simulink model "LKAS_AutoSave_20200908_1055"  (R2018b)
settings: Solver=FixedStepDiscrete  StartTime=0.0  StopTime=10.0  FixedStep=0.01  RelTol=1e-3
InitFcn:
  | tmpVer = ver('MATLAB');
  | tmpVer = str2num(tmpVer.Version);
  | % -------------------------------------------------------------------
  | %  MATLAB file generated by Simulink.saveVars on 21-Nov-2019 10:06:14
  | %  MATLAB version: 7.13.0.564 (R2011b)
  | % -------------------------------------------------------------------
  | 
  | 
  | SInt16 = Simulink.AliasType;
  | SInt16.Description = 'Num';
  | if (tmpVer > 7.11)
  | 	SInt16.DataScope = 'Auto';
  | end
  | SInt16.HeaderFile = 'Rte_Type.h';
  | SInt16.BaseType = 'int16';
  | 
  | SInt32 = Simulink.AliasType;
  | SInt32.Description = 'Num';
  | if (tmpVer > 7.11)
  | 	SInt32.DataScope = 'Auto';
  | end
  | SInt32.HeaderFile = 'Rte_Type.h';
  | SInt32.BaseType = 'int32';
  | 
  | SInt8 = Simulink.AliasType;
  | SInt8.Description = 'Num';
  | if (tmpVer > 7.11)
  | 	SInt8.DataScope = 'Auto';
  | end
  | SInt8.HeaderFile = 'Rte_Type.h';
  | SInt8.BaseType = 'int8';
  | 
  | T_A_m2_1024_1_u32 = Simulink.NumericType;
  | T_A_m2_1024_1_u32.Description = 'm2 (square meters  (m2))';
  | if (tmpVer > 7.11)
  | 	T_A_m2_1024_1_u32.DataScope = 'Auto';
  | end
  | T_A_m2_1024_1_u32.HeaderFile = 'Rte_Type.h';
  | T_A_m2_1024_1_u32.DataTypeMode = 'Fixed-point: slope and bias scaling';
  | T_A_m2_1024_1_u32.SignednessBool = false;
  | T_A_m2_1024_1_u32.WordLength = 32;
  | T_A_m2_1024_1_u32.FixedExponent = -10;
  | T_A_m2_1024_1_u32.SlopeAdjustmentFactor = 1;
  | T_A_m2_1024_1_u32.Bias = 0;
  | T_A_m2_1024_1_u32.DataTypeOverride = 'Inherit';
  | T_A_m2_1024_1_u32.IsAlias = true;
  | 
  | T_A_m2_65536_1_u16 = Simulink.NumericType;
  | T_A_m2_65536_1_u16.Description = 'm2 (square meters  (m2))';
  | if (tmpVer > 7.11)
  | 	T_A_m2_65536_1_u16.DataScope = 'Auto';
  | end
  | T_A_m2_65536_1_u16.HeaderFile = 'Rte_Type.h';
  | T_A_m2_65536_1_u16.DataTypeMode = 'Fixed-point: slope and bias scaling';
  | T_A_m2_65536_1_u16.SignednessBool = false;
  | T_A_m2_65536_1_u16.WordLength = 16;
  | T_A_m2_65536_1_u16.FixedExponent = -16;
  | T_A_m2_65536_1_u16.SlopeAdjustmentFactor = 1;
  | T_A_m2_65536_1_u16.Bias = 0;
  | T_A_m2_65536_1_u16.DataTypeOverride = 'Inherit';
  | ... (+4598 lines)
StopFcn:
  | clear  T_A_m2_1024_1_u32 T_A_m2_65536_1_u16 T_A_m2_Float32 T_A_mm2_10_1_u16 T_A_mm2_4_1_s16 T_A_mm2_Float32 T_Cnt_Num_10_1_u32 T_Cnt_Num_1_1_s16 T_Cnt_Num_1_1_s32 T_Cnt_Num_1_1_s8 T_Cnt_Num_1_1_u16 T_Cnt_Num_1_1_u32 T_Cnt_Num_1_1_u8 T_E_J_1_1_s32 T_E_J_Float32 T_E_kJ_128_1_s32 T_E_kJ_Float32 T_E_kwh_10_1_u16 T_E_kwh_Float32 T_Epl_kwhpkm_100_1_u16 T_Epl_kwhpkm_Float32 T_F_N_1_1_s16 T_F_N_Float32 T_I_A_1000_1_u16 T_I_A_1048576_1_s32 T_I_A_2048_1_s16 T_I_A_32_1_s16 T_I_A_Float32 T_I_mA_1_1_s16 T_I_mA_32768_128_s16 T_I_mA_Float32 T_J_kgpm2_128_1_u16 T_J_kgpm2_Float32 T_K_NA_1000_1_s16 T_K_NA_100_1_s16 T_K_NA_100_1_u16 T_K_NA_1024_1_s16 T_K_NA_1024_1_u16 T_K_NA_128_1_s16 T_K_NA_128_1_u16 T_K_NA_128_1_u8 T_K_NA_16777216_1_u32 T_K_NA_16_1_s16 T_K_NA_16_1_u16 T_K_NA_16_1_u8 T_K_NA_1_16_u16 T_K_NA_1_1_s16 T_K_NA_1_1_u16 T_K_NA_1_1_u8 T_K_NA_32768_1_s16 T_K_NA_32768_1_u16 T_K_NA_32_1_s8 T_K_NA_4096_1_u16 T_K_NA_4194304_1_s32 T_K_NA_4194304_1_u16 T_K_NA_65536_1_s32 T_K_NA_65536_1_u16 T_K_NA_8192_1_s16 T_K_NA_8_1_s16 T_K_NA_Float32 T_M_Nm_16_1_s16 T_M_Nm_1_1_s16 T_M_Nm_32768_1_s16 T_M_Nm_32_1_s16 T_M_Nm_4_1_s16 T_M_Nm_512_1_s16 T_M_Nm_Float32 T_P_W_1_4_s16 T_P_W_1_8_s16 T_P_W_Float32 T_P_kW_128_1_s16 T_P_kW_1_8_s16 T_P_kW_8_1_s32 T_P_kW_Float32 T_Pct_pct_1024_1_s32 T_Pct_pct_1024_1_u32 T_Pct_pct_10_1_s16 T_Pct_pct_10_1_u32 T_Pct_pct_128_100_s8 T_Pct_pct_1_1_s16 T_Pct_pct_1_4_u8 T_Pct_pct_255_100_u16 T_Pct_pct_255_100_u8 T_Pct_pct_256_1_s16 T_Pct_pct_256_1_u16 T_Pct_pct_65535_100_u16 T_Pct_pct_Float32 T_R_ohm_1024_1_s16 T_R_ohm_32_1_s16 T_R_ohm_Float32 T_TK_K_16_1_s16 T_TK_K_Float32 T_T_degC_10_400_1_u16 T_T_degC_16_1_s16 T_T_degC_1_40_1_u8 T_T_degC_2_80_1_u8 T_T_degC_Float32 T_U_V_1000_1_u16 T_U_V_10_1_u8 T_U_V_200_1_u8 T_U_V_32_1_s16 T_U_V_4096_1_s16 T_U_V_512_1_s16 T_U_V_65535_8_u16 T_U_V_8192_1_u16 T_U_V_Float32 T_U_mV_1_1_s16 T_U_mV_256_20_u16 T_U_mV_Float32 T_V_l_256_1_s16 T_V_l_4096_1_s16 T_V_l_64_1_s16 T_V_l_65535_100_u16 T_V_l_Float32 T_V_ml_128_1_s16 T_V_ml_1_1_s16 T_V_ml_32768_1_s16 T_V_ml_Float32 T_V_ul_32_1_u16 T_V_ul_Float32 T_Vpl_clpkm_512_1_u16 T_Vpl_clpkm_Float32 T_a_kphps_16_1_s16 T_a_kphps_Float32 T_a_mps2_128_1_s16 T_a_mps2_Float32 T_c_MJpkg_256_1_s16 T_c_MJpkg_Float32 T_c_kJpgpK_1024_1_s16 T_c_kJpgpK_Float32 T_c_kJpkgpK_128_1_u16 T_c_kJpkgpK_Float32 T_chrg_Ah_1_1_s16 T_chrg_Ah_1_1_u16 T_chrg_Ah_1_1_u8 T_chrg_Ah_256_1_u16 T_chrg_Ah_4194304_1_s32 T_chrg_Ah_512_1_u16 T_chrg_Ah_8_1_u16 T_chrg_Ah_Float32 T_cmp_NA_100_1_s16 T_cmp_NA_128_1_s16 T_cmp_NA_16_1_s16 T_cmp_NA_32768_1_u16 T_cmp_NA_Float32 T_d2n_rpmps2_4_1_s16 T_d2n_rpmps2_Float32 T_dPct_pctps_16_1_s16 T_dPct_pctps_256_1_s16 T_dPct_pctps_Float32 T_dT_degCps_128_1_s16 T_dT_degCps_Float32 T_dV_lph_1_1_s16 T_dV_lph_Float32 T_dV_lpm_128_1_s16 T_dV_lpm_32_1_s16 T_dV_lpm_Float32 T_dV_lps_1024_1_u16 T_dV_lps_4_1_u16 T_dV_lps_Float32 T_dV_mlps_1024_1_s16 T_dV_mlps_Float32 T_d_BitField16 T_dm_gps_128_1_s16 T_dm_gps_128_1_u16 T_dm_gps_256_1_u16 T_dm_gps_Float32 T_dm_mgps_1_1_s16 T_dm_mgps_Float32 T_dn_rpmps_1_1_s16 T_dn_rpmps_2_1_s16 T_dn_rpmps_Float32 T_dp_Paps_1_1_s16 T_dp_Paps_Float32 T_dp_kPaps_1_1_s16 T_dp_kPaps_8_1_s16 T_dp_kPaps_Float32 T_dphi_degps_128_1_s16 T_dphi_degps_8_1_s16 T_dphi_degps_Float32 T_dr_ps_256_1_s16 T_dr_ps_Float32 T_drho_mgplps_1_2_s16 T_drho_mgplps_Float32 T_e_NA_1_1_u8 T_f_Hz_1_1_u16 T_f_Hz_1_1_u32 T_f_Hz_64_1_u16 T_f_Hz_8_1_s16 T_f_Hz_Float32 T_g_BitField32 T_l_km_16_1_s16 T_l_km_1_1_u16 T_l_km_1_1_u32 T_l_km_Float32 T_l_m_1024_1_s16 T_l_m_16_1_s16 T_l_m_1_1_u32 T_l_m_Float32 T_l_mm_16_1_s16 T_l_mm_1_1_u16 T_l_mm_4096_1_s16 T_l_mm_4_1_u8 T_l_mm_64_1_s16 T_l_mm_Float32 T_m_g_1_1_s16 T_m_g_2048_1_s16 T_m_g_32_1_u16 T_m_g_Float32 T_m_kg_1024_1_s16 T_m_kg_1_1_s16 T_m_kg_1_1_u32 T_m_kg_Float32 T_m_mg_128_1_s16 T_m_mg_32_1_s16 T_m_mg_Float32 T_n_rpm_1_1_s16 T_n_rpm_1_25_u8 T_n_rpm_256_50_u16 T_n_rpm_2_25_u8 T_n_rpm_4_1_u16 T_n_rpm_Float32 T_p_MPa_64_1_s16 T_p_MPa_Float32 T_p_Pa_1_1_s16 T_p_Pa_Float32 T_p_kPa_1_10_u16 T_p_kPa_1_1_s16 T_p_kPa_1_1_u8 T_p_kPa_256_1_u16 T_p_kPa_32_1_u16 T_p_kPa_64_1_s16 T_p_kPa_Float32 T_phi_deg_100_1_s16 T_phi_deg_1024_1_s16 T_phi_deg_128_1_s16 T_phi_deg_1_1_u8 T_phi_deg_256_1_s16 T_phi_deg_2_1_s8 T_phi_deg_32_1_s16 T_phi_deg_512_6_s32 T_phi_deg_Float32 T_phi_rad_2048_1_s16 T_phi_rad_Float32 T_r_NA_1024_1_s16 T_r_NA_1024_1_u16 T_r_NA_16384_1_s16 T_r_NA_16_1_s16 T_r_NA_256_1_s8 T_r_NA_256_1_u16 T_r_NA_32768_1_u16 T_r_NA_32_1_u16 T_r_NA_4096_1_s16 T_r_NA_65535_2_u16 T_r_NA_8192_1_u16 T_r_NA_Float32 T_rho_gpl_8192_1_s16 T_rho_gpl_Float32 T_rho_kgpm3_16_1_s16 T_rho_kgpm3_Float32 T_rho_mgpl_1_1_s16 T_rho_mgpl_64_1_s16 T_rho_mgpl_Float32 T_t_hour_1_1_s16 T_t_hour_Float32 T_t_m_1_1_u16 T_t_m_Float32 T_t_ms_1_1_s16 T_t_ms_1_1_u16 T_t_ms_1_1_u32 T_t_ms_4096_1_s16 T_t_ms_64_1_s16 T_t_ms_Float32 T_t_s_1000_1_s16 T_t_s_100_1_s16 T_t_s_10_1_s16 T_t_s_10_1_u16 T_t_s_1_1_s16 T_t_s_1_1_u16 T_t_s_1_1_u32 T_t_s_Float32 T_t_us_10_1_u32 T_t_us_1_1_s16 T_t_us_1_1_u32 T_t_us_1_4_u16 T_t_us_Float32 T_v_kph_1_1_u8 T_v_kph_64_1_s16 T_v_kph_64_1_u16 T_v_kph_Float32 T_v_mps_256_1_s16 T_v_mps_Float32 T_w_radps_32_1_s16 T_w_radps_Float32 T_y_BitField8 T_y_BitFieldDiagProgress T_y_BitFieldDiagStatus T_y_NA_1_1_u8 SInt16 SInt32 SInt8 T_BOOLEAN UInt16 UInt32 UInt8 s16 s32 s8 u16 u32 u8
model workspace (MAT data in the model file):
  MCOS : class17 (value not decoded)
  MCOS : class17 (value not decoded)
  MCOS : class17 (value not decoded)
  MCOS : class17 (value not decoded)
  MCOS : class17 (value not decoded)
  MCOS : class17 (value not decoded)
  MCOS : class17 (value not decoded)
  MCOS : class17 (value not decoded)
  MCOS : class17 (value not decoded)
  MCOS : class17 (value not decoded)
  MCOS : class17 (value not decoded)
  MCOS : class17 (value not decoded)
  MCOS : class17 (value not decoded)
  MCOS : class17 (value not decoded)
  MCOS : class17 (value not decoded)
  MCOS : class17 (value not decoded)
  MCOS : class17 (value not decoded)
  MCOS : class17 (value not decoded)
  MCOS : class17 (value not decoded)
  MCOS : class17 (value not decoded)
  MCOS : class17 (value not decoded)
  MCOS : class17 (value not decoded)
  MCOS : class17 (value not decoded)
  MCOS : class17 (value not decoded)
  MCOS : class17 (value not decoded)
  MCOS : class17 (value not decoded)
  MCOS : class17 (value not decoded)
  MCOS : class17 (value not decoded)
  MCOS : class17 (value not decoded)
  MCOS : class17 (value not decoded)
  MCOS : class17 (value not decoded)
  MCOS : class17 (value not decoded)
  MCOS : class17 (value not decoded)
  MCOS : class17 (value not decoded)
  MCOS : class17 (value not decoded)
  MCOS : class17 (value not decoded)
  MCOS : class17 (value not decoded)
  MCOS : class17 (value not decoded)
  MCOS : class17 (value not decoded)
  MCOS : class17 (value not decoded)
  MCOS : class17 (value not decoded)
  MCOS : class17 (value not decoded)
  MCOS : class17 (value not decoded)
  MCOS : class17 (value not decoded)
  MCOS : class17 (value not decoded)
  MCOS : class17 (value not decoded)
  MCOS : class17 (value not decoded)
  MCOS : class17 (value not decoded)
  MCOS : class17 (value not decoded)
  MCOS : class17 (value not decoded)
  MCOS : class17 (value not decoded)
  MCOS : class17 (value not decoded)
  MCOS : class17 (value not decoded)
  MCOS : class17 (value not decoded)
  MCOS : class17 (value not decoded)
  MCOS : class17 (value not decoded)
  MCOS : class17 (value not decoded)
  MCOS : class17 (value not decoded)
  MCOS : class17 (value not decoded)
  MCOS : class17 (value not decoded)
  MCOS : class17 (value not decoded)
  MCOS : class17 (value not decoded)
  MCOS : class17 (value not decoded)
  MCOS : class17 (value not decoded)
  MCOS : class17 (value not decoded)
  MCOS : class17 (value not decoded)
  MCOS : class17 (value not decoded)
  MCOS : class17 (value not decoded)
  MCOS : class17 (value not decoded)
  MCOS : class17 (value not decoded)
  MCOS : class17 (value not decoded)
  MCOS : class17 (value not decoded)
  MCOS : class17 (value not decoded)
  MCOS : class17 (value not decoded)
  MCOS : class17 (value not decoded)
  MCOS : class17 (value not decoded)
  MCOS : class17 (value not decoded)
  MCOS : class17 (value not decoded)
  MCOS : class17 (value not decoded)
  MCOS : class17 (value not decoded)
  MCOS : class17 (value not decoded)
  MCOS : class17 (value not decoded)
  MCOS : class17 (value not decoded)
  MCOS : class17 (value not decoded)
  MCOS : class17 (value not decoded)
  MCOS : class17 (value not decoded)
  MCOS : class17 (value not decoded)
  MCOS : class17 (value not decoded)
  MCOS : class17 (value not decoded)
undefined symbols (not defined in the file): LKA_CarWidth, LKA_SampleTime, LKA_StrRatio_C, LKA_Veh2CamL_C, LKA_Veh2CamW_C, LKA_WhlBaseL_C, LL_CompSWA_C, LL_CrvtPrvwT_C, LL_DesDvt_C, LL_DvtComp_C, LL_DvtPrvwT_C, LL_DvtSpdDet_vDvtSpdMin_C, LL_HdAgExT_C, LL_HdAgPrvwT_C, LL_LAccMax_C, LL_LAccRMax_C, LL_LDW_EarliestWarnLine_C, LL_LDW_LatestWarnLine_C, LL_LDWS_SUPPRESS_HEADING, LL_LFClb_TFC_DiffCtlBalance, LL_LFClb_TFC_DiffCtrlMaxSWA, LL_LFClb_TFC_DiffCtrlRatio, LL_LFClb_TFC_facmGainLutGain1_C, LL_LFClb_TFC_facmGainLutGain2_C, LL_LFClb_TFC_facmIntegRatio, LL_LFClb_TFC_facmKlat_C, LL_LFClb_TFC_FfCtlRatio_C, LL_LFClb_TFC_phiIntegCtlMaxSWA_C, LL_LFClb_TFC_tiKlatPrvwT_C, LL_LFClb_TFC_vGainLutVehSpdLwr_C, LL_LFClb_TFC_vGainLutVehSpdUpr_C, LL_LKA_EarliestWarnLine_C, LL_LKA_LatestWarnLine_C, LL_LKAExPrcs_ExitC0Dvt, LL_LKAExPrcs_ExitC0Swt, LL_LKAExPrcs_tiExitTime1, LL_LKAExPrcs_tiExitTime2, LL_LKAExPrcs_tiExitTime3, LL_LKAS_OUT_OF_CONTROL_LAT_VEL, LL_LKAS_OUT_OF_CONTROL_TTLC, LL_LKASWASyn_M0, LL_LKASWASyn_M1, LL_LKASWASyn_M2, LL_LKASWASyn_M3K, LL_LKASWASyn_SWAaddMax, LL_LKASWASyn_T2, LL_LKASWASyn_tiTrqSwaRtTime, LL_LKASWASyn_tiTrqSwaTime, LL_LKASWASyn_TrqMax, LL_LKASWASyn_TrqSwaAddSwt, LL_LKASWASyn_TrqSwaRateDiff, LL_LSpdCompT_C, LL_lStpLngth_C, LL_MAX_DELAY_EPSSTAR_TIME, LL_MAX_DRIVER_TORQUE_DISABLE, LL_MAX_DRIVER_TORQUE_ENABLE, LL_MAX_LANE_WIDTH_DISABLE, LL_MAX_LANE_WIDTH_ENABLE, LL_MAX_LAT_ACC_DISABLE, LL_MAX_LAT_ACC_ENABLE ... (+29)
libraries: simulink x134, dspstat3 x3, simulink_extras x1
(part 6 of 19)

== system LKAS_AutoSave_20200908_1055/LKAS/LL/LL Inputs Mapping/bsVehMovInfo ==
  bsVehMovInfoIn : Inport
  Bus Creator : BusCreator  Inputs=10
  Bus Selector2 : BusSelector  OutputSignals=ESC_LatAcc,ESC_LatAcc_Valid,ESC_YawRate,ESC_YawRate_Valid,ESC_UnYawRate,ESC_VehSpd,ESC_LonAcc,ESC_LonAcc_Valid,ESC_Brake_Press,ESC_VehSpd_Valid
  bsVehMovInfoOut : Outport
  wires:
  Bus Creator/1 -> bsVehMovInfoOut/1
  Bus Selector2/10 -> Bus Creator/10  "<ESC_VehSpd_Valid>"
  Bus Selector2/9 -> Bus Creator/9  "<ESC_Brake_Press>"
  Bus Selector2/8 -> Bus Creator/8  "<ESC_LonAcc_Valid>"
  Bus Selector2/7 -> Bus Creator/7  "<ESC_LonAcc>"
  Bus Selector2/6 -> Bus Creator/6  "<ESC_VehSpd>"
  Bus Selector2/5 -> Bus Creator/5  "<ESC_UnYawRate>"
  Bus Selector2/4 -> Bus Creator/4  "<ESC_YawRate_Valid>"
  Bus Selector2/3 -> Bus Creator/3  "<ESC_YawRate>"
  Bus Selector2/2 -> Bus Creator/2  "<ESC_LatAcc_Valid>"
  Bus Selector2/1 -> Bus Creator/1  "<ESC_LatAcc>"
  bsVehMovInfoIn/1 -> Bus Selector2/1

== system LKAS_AutoSave_20200908_1055/LKAS/LL/LLOn/LDW ==
  LDW_stLDWActvFlg : Inport
  LDW_bsInInfoSyn : Inport  Port=2
  LDW_bsLDWClb : Inport  Port=3
  states : EnablePort  StatesWhenEnabling=reset
      settings: AttributesFormatString=states = %<StatesWhenEnabling>
  Bus Selector : BusSelector  OutputSignals=bsLaneInfo.bsL0Info.L0_C1,bsLaneInfo.bsR0Info.R0_C1
  Bus Selector1 : BusSelector  OutputSignals=LL_LDWS_SUPPRESS_HEADING
  Heading Angle Detection (HdAgDet) : Subsystem  Description=|
      | Block Name: Heading Angle Detection
      | Ab.: HdAgDet
      | No.: 1.3.1.0
      | Rev: 0.0.1
      | Update Date: 19-3-26
  LDWWarnInfo : MATLAB Function  TreatAsAtomicUnit=on
  LDW_Flag : Outport  OutputWhenDisabled=reset  InitialOutput=0
  wires:
  LDW_bsInInfoSyn/1 -> Bus Selector/1
  LDW_stLDWActvFlg/1 -> Heading Angle Detection (HdAgDet)/1(HdAgDet_stLDWActvFlg), LDWWarnInfo/1(LDW_stLDWActvFlg)
  Bus Selector/1 -> Heading Angle Detection (HdAgDet)/2(HdAgDet_phiHdAgLft)  "<L0_C1>"
  Bus Selector/2 -> Heading Angle Detection (HdAgDet)/3(HdAgDet_phiHdAgRgt)  "<R0_C1>"
  LDW_bsLDWClb/1 -> Bus Selector1/1
  Bus Selector1/1 -> Heading Angle Detection (HdAgDet)/4(HdAgDet_phiHdAgThres_C)  "<LL_LDWS_SUPPRESS_HEADING>"
  Heading Angle Detection (HdAgDet)/1(HdAgDet_stHdAgDetFlg) -> LDWWarnInfo/2(LDW_stHdAgDetFlg)
  LDWWarnInfo/1(LDWWarnInfo) -> LDW_Flag/1

== system LKAS_AutoSave_20200908_1055/LKAS/LL/LLOn/LKA ==
  LKA_bsInInfoSyn : Inport
  LKA_bsLKAInPInfo : Inport  Port=2
  LKA_bsLKAClb : Inport  Port=3
  LKA_bsConstantClb : Inport  Port=4
  states = reset : EnablePort  StatesWhenEnabling=reset  ShowOutputPort=on
  Bus Selector : BusSelector  OutputSignals=LKA_SampleTime
  Cast To Single : DataTypeConversion  OutDataTypeStr=uint8
  Driver Torque Addition (DTA) : Subsystem
  LKA Exit Processing (LKAExPrcs) : Subsystem  Description=|
      | Block Name: LKA Exit Processing 
      | Ab.: LKAExPrcs
      | No.: 1.2.2.0
      | Rev: 0.0.1
      | Update Date: 19-5-13
  "LKA Motion Planning (LKAMP) " : Subsystem  Description=|
      | Block Name: LKA Motion Planning
      | Ab.: LKAMP
      | No.: 1.2.3.0
      | Rev: 0.0.1
      | Update Date: 19-5-13
  LKA SWA Limit (LKASWALim) : Subsystem  Description=|
      | Block Name: LKA SWA Synthesis
      | Ab.: LKASWASyn
      | No.: 1.2.6.0
      | Rev: 0.0.1
      | Update Date: 19-5-13
  LKA_Mon : Subsystem
  Lane Following (LF) : Subsystem  Description=|
      | Block Name: Lane Following
      | Ab.: LF
      | No.: 02
      | Rev: 00.00.01
      | Update Date: 19-3-28
  Plan To LaneFollowing (PTLF) : Subsystem
  LKA_ExitFlg : Outport  OutputWhenDisabled=reset  InitialOutput=0
  LKA_phiSWACmd : Outport  Port=2  OutputWhenDisabled=reset  InitialOutput=0
  LKA_M : Outport  Port=3  OutputWhenDisabled=reset  InitialOutput=0
  LKAMon : Outport  Port=4  OutputWhenDisabled=reset  InitialOutput=0
  tag scope: ActFlg=global, Ff=global, LKA_ConstantClb=global, LKA_ExitFlg_Mon=global, LKA_SampleTime=global, PT1=global
  wires:
  Bus Selector/1 -> [LKA_SampleTime]  "<LKA_SampleTime>"
  LKA_bsConstantClb/1 -> Bus Selector/1, [LKA_ConstantClb]
  Cast To Single/1 -> [ActFlg]  "ActFlg"
  Plan To LaneFollowing (PTLF)/1(SWACmd) -> LKA SWA Limit (LKASWALim)/1(LKASWALim_phiTFCSWACmd)  "PTLFSWACmd"
  states = reset/1 -> Cast To Single/1
  LKA SWA Limit (LKASWALim)/1(LKASWALim_phiSWACmd) -> LKA_phiSWACmd/1  "phiSWACmd"
  LKA Exit Processing (LKAExPrcs)/1(LKAExPrcs_stExFlg) -> [LKA_ExitFlg_Mon], LKA_ExitFlg/1
  [Ff] -> Plan To LaneFollowing (PTLF)/5(Ff)
  [P] -> Plan To LaneFollowing (PTLF)/6(P)
  [I] -> Plan To LaneFollowing (PTLF)/7(I)
  [D] -> Plan To LaneFollowing (PTLF)/8(D)
  Driver Torque Addition (DTA)/1(DTA_phiDTASWACmd) -> [DT]  "DT"
  [DT] -> Plan To LaneFollowing (PTLF)/4(DrvTrq)
  [Plan] -> Plan To LaneFollowing (PTLF)/2(Plan)
  [PT1] -> Plan To LaneFollowing (PTLF)/3(T1)
  [PT1] -> LKA Exit Processing (LKAExPrcs)/4(LKAExPrcs_PlanT1)
  [ActFlg] -> "LKA Motion Planning (LKAMP) "/2(LKAMP_stLKAActvFlg)
  [LKA_ConstantClb] -> "LKA Motion Planning (LKAMP) "/5(LLClb_bsConstantClb)
  [LKA_ConstantClb] -> Lane Following (LF)/4(LF_bsConstantClb)
  LKA_bsLKAInPInfo/1 -> [LKAInPInfo]
  [LKAInPInfo] -> "LKA Motion Planning (LKAMP) "/3(LKAMP_bsLKAInPInfo)
  [LKAInPInfo] -> LKA Exit Processing (LKAExPrcs)/2(LKAExPrcs_bsLKAInPInfo)
  [LKAInPInfo] -> Plan To LaneFollowing (PTLF)/1(InP)
  LKA_bsLKAClb/1 -> [LKA_bsLKAClb]
  [LKAInPInfo] -> LKA SWA Limit (LKASWALim)/3(LKASWALim_bsLKAInPInfo)
  [LKA_bsLKAClb] -> LKA Exit Processing (LKAExPrcs)/3(LKAExPrcs_bsLKAClb)
  [LKA_bsLKAClb] -> "LKA Motion Planning (LKAMP) "/4(LKAMP_bsLKAClb)
  [LKA_bsLKAClb] -> Driver Torque Addition (DTA)/2(DTA_bsLFClb)
  [LKA_bsLKAClb] -> Lane Following (LF)/3(LF_bsLFClb)
  [LKA_bsLKAClb] -> LKA SWA Limit (LKASWALim)/4(LKASWALim_bsLKAClb)
  LKA_bsInInfoSyn/1 -> [LKA_bsInInfoSyn]
  [LKA_bsInInfoSyn] -> LKA Exit Processing (LKAExPrcs)/1(LKAExPrcs_bsInInfoSyn)
  [LKA_bsInInfoSyn] -> "LKA Motion Planning (LKAMP) "/1(LKAMP_bsInInfoSyn)
  [LKA_bsInInfoSyn] -> Driver Torque Addition (DTA)/1(DTA_bsInInfoSyn)
  [LKA_bsInInfoSyn] -> Lane Following (LF)/1(LF_bsInInfoSyn)
  [Ff] -> LKA SWA Limit (LKASWALim)/2(LKASWALim_Ff)
  [LKAInPInfo] -> Lane Following (LF)/2(LF_bsLKAInPInfo)
  Driver Torque Addition (DTA)/2(DTA_M) -> LKA_M/1
  Lane Following (LF)/3(LF_phiIntegSWACmd) -> [I]
  Lane Following (LF)/1(LF_phiFfLFSWACmd) -> [Ff]
  Lane Following (LF)/2(LF_phiPropSWACmd) -> [P]
  Lane Following (LF)/4(LF_phiDiffSWACmd) -> [D]
  "LKA Motion Planning (LKAMP) "/1(LKAMP_phiSWACmd) -> [Plan]  "PlanSWACmd"
  "LKA Motion Planning (LKAMP) "/3(LKAMP_tiT2) -> ?  "PlanT2"
  "LKA Motion Planning (LKAMP) "/2(LKAMP_tiT1) -> [PT1]  "PlanT1"
  LKA_Mon/1(LKAMon) -> LKAMon/1

== system LKAS_AutoSave_20200908_1055/LKAS/LL/LLOn/LKA Input Processing (LKAInP) ==
  LKAInP_stLKAActvFlg : Inport
  LKAInP_bsInInfoSyn : Inport  Port=2
  LKAInP_bsLKAClb : Inport  Port=3
  Bus Creator : BusCreator  Inputs=6
  Bus Creator1 : BusCreator  Inputs=3
  Delay : Delay  DelayLength=1
  Lane Width Calculation (LW) : Subsystem
  Predicted Deviation Calculation (PrDvt) : Subsystem
  Predicted Heading Angle Calculation (PrHdAg) : Subsystem
  Previewed Curvature (PrCrvt) : Subsystem
  Steering Wheel Position Calculation (SWAPosCal) : Subsystem
  TTLC Calculation (TTLCCalc) : Subsystem  Description=|
      | Block Name: TTLC Calculation
      | Ab.: TTLCCalc
      | No.: 1.1.1.1
      | Rev: 0.0.1
      | Update Date: 19-3-26
  Under The Limit (UndrLim) : Subsystem
  LKAInP_bsLKAInPInfo : Outport
  wires:
  Delay/1 -> Previewed Curvature (PrCrvt)/1(PrvwCrvt_stLKAActvFlg), Predicted Heading Angle Calculation (PrHdAg)/2(PrdcHdAg_stLKAActvFlg), Predicted Deviation Calculation (PrDvt)/1(PrdcDvt_stLKAActvFlg)
  LKAInP_bsInInfoSyn/1 -> Steering Wheel Position Calculation (SWAPosCal)/1(SWAPosCal_bsInInfoSyn), Under The Limit (UndrLim)/1(UndrLim_bsInInfoSyn), Previewed Curvature (PrCrvt)/2(PrvwCrvt_bsInInfoSyn), Predicted Heading Angle Calculation (PrHdAg)/3(PrHdAg_bsInInfoSyn), Predicted Deviation Calculation (PrDvt)/2(PrdcDvt_bsInInfoSyn), TTLC Calculation (TTLCCalc)/1(bsInfo), Lane Width Calculation (LW)/1(LW_bsInInfoSyn)
  Bus Creator/1 -> LKAInP_bsLKAInPInfo/1
  LKAInP_bsLKAClb/1 -> Under The Limit (UndrLim)/2(UndrLim_bsUndrLimClb), Previewed Curvature (PrCrvt)/3(PrvwCrvt_tiCrvtPrvwT_C), Predicted Heading Angle Calculation (PrHdAg)/4(PrHdAg_bsLKAClb), Predicted Deviation Calculation (PrDvt)/4(PrdcDvt_bsLKAClb)
  Predicted Heading Angle Calculation (PrHdAg)/1(PrHdAg_bsPrHdAgInfo) -> Predicted Deviation Calculation (PrDvt)/3(PrdcDvt_bsPrdcHdAgInfo), Bus Creator1/2  "bsPrHdAgInfo"
  Predicted Deviation Calculation (PrDvt)/1(PrdcDvt_bsPrdcDvtInfo) -> TTLC Calculation (TTLCCalc)/2(bsPrDvtInfo), Bus Creator1/1  "bsPrDvtInfo"
  Previewed Curvature (PrCrvt)/1(PrvwCrvt_bsPrvwCrvtInfo) -> TTLC Calculation (TTLCCalc)/3(bsPrvwCrvtInfo), Bus Creator1/3  "bsPrCrvtInfo"
  Bus Creator1/1 -> Bus Creator/3  "Pr_bsPrInfo"
  Under The Limit (UndrLim)/1(UndrLim_phiSWAMax) -> Bus Creator/4  "UndrLim_phiSWAMax"
  Under The Limit (UndrLim)/2(UndrLim_dphiSWARMax) -> Bus Creator/5  "UndrLim_dphiSWARMax"
  LKAInP_stLKAActvFlg/1 -> Delay/1
  Steering Wheel Position Calculation (SWAPosCal)/1(SWAPosCal) -> Bus Creator/6  "LKAInP_phiSWAPos"
  Lane Width Calculation (LW)/1(LW_LaneWidth) -> Bus Creator/1  "LW_LaneWidth"
  TTLC Calculation (TTLCCalc)/1(TTLCCalc_bsTTLCInfo) -> Bus Creator/2, Predicted Heading Angle Calculation (PrHdAg)/1(PrHdAg_bsTTLCInfo)  "TTLC_bsTTLCInfo"

== system LKAS_AutoSave_20200908_1055/LKAS/LL/LLOn/LL State Determination (LLStateDet) ==
  LLStateDet_stDACMode : Inport
  LLStateDet_bsInInfoSyn : Inport  Port=2
  LLStateDet_bsLKAInPInfo : Inport  Port=3
  LLStateDet_bsLLSMConClb : Inport  Port=4
  LLStateDet_stExitFlg : Inport  Port=5
  LLStateDet_SignalFault : Inport  Port=6
  Bus Creator : BusCreator  Inputs=3
  Delay : Delay  DelayLength=1
  Delay1 : Delay  DelayLength=1
  LDW_State_Machine : Stateflow chart  Description=|  TreatAsAtomicUnit=on
      | Block Name: LDW State Machine
      | Ab.: LDWSM
      | No.: 1.1.2.0
      | Rev: 0.0.1
      | Update Date: 19-3-26
      settings: RTWSystemCode=Nonreusable function
  LKA_State_Machine : Stateflow chart  Description=|  TreatAsAtomicUnit=on
      | Block Name: LKA State Machine
      | Ab.: LKASM
      | No.: 1.1.3.0
      | Rev: 0.0.1
      | Update Date: 19-3-26
      settings: RTWSystemCode=Nonreusable function
  LL State Machine Conditions (LLSMCon) : Subsystem
  LLStateDet_bsLLState : Outport
  LLStateDet_stLDWActvFlg : Outport  Port=2
  LLStateDet_stLKAActvFlg : Outport  Port=3
  tag scope: LDW_State_Mon=global, LKA_State_Mon=global
  wires:
  LL State Machine Conditions (LLSMCon)/2(LLSMCon_stLDWEnaCSyn) -> LDW_State_Machine/2(LDWSM_stEnaCSyn)
  LL State Machine Conditions (LLSMCon)/3(LLSMCon_stLDWDisblCSyn) -> LDW_State_Machine/3(LDWSM_stDisblCSyn)
  LL State Machine Conditions (LLSMCon)/4(LLSMCon_stLDWActvCSyn) -> LDW_State_Machine/4(LDWSM_stActvCSyn)
  LL State Machine Conditions (LLSMCon)/5(LLSMCon_stLDWDeactvCSyn) -> LDW_State_Machine/5(LDWSM_stDeactvCSyn)
  LL State Machine Conditions (LLSMCon)/1(LLSMCon_stDACMode) -> LKA_State_Machine/1(LKASM_stLMCMode), Bus Creator/2, LDW_State_Machine/1(LDWSM_stLMCMode)  "DACMode"
  LDW_State_Machine/1(LDWSM_stLDWActvFlg) -> LLStateDet_stLDWActvFlg/1
  LKA_State_Machine/1(LKASM_stLKAActvFlg) -> LLStateDet_stLKAActvFlg/1
  Delay1/1 -> LL State Machine Conditions (LLSMCon)/5(LLSMCon_bsLLState)
  Bus Creator/1 -> Delay1/1, LLStateDet_bsLLState/1  "LLState"
  LKA_State_Machine/2(LKASM_stLKAState) -> [LKA_State_Mon], Bus Creator/3  "LKA_State"
  LDW_State_Machine/2(LDWSM_stLDWState) -> [LDW_State_Mon], Bus Creator/1  "LDW_State"
  LL State Machine Conditions (LLSMCon)/6(LLSMCon_stLDWFaultCSyn) -> LDW_State_Machine/6(LDWSM_stFaultCSyn)
  LL State Machine Conditions (LLSMCon)/7(LLSMCon_stLKAEnaCSyn) -> LKA_State_Machine/2(LKASM_stEnaCSyn)
  LL State Machine Conditions (LLSMCon)/8(LLSMCon_stLKADisblCSyn) -> LKA_State_Machine/3(LKASM_stDisblCSyn)
  LL State Machine Conditions (LLSMCon)/9(LLSMCon_stLKAActvCSyn) -> LKA_State_Machine/4(LKASM_stActvCSyn)
  LL State Machine Conditions (LLSMCon)/10(LLSMCon_stLKADeactvCSyn) -> LKA_State_Machine/5(LKASM_stDeactvCSyn)
  LL State Machine Conditions (LLSMCon)/11(LLSMCon_stLKAFaultCSyn) -> LKA_State_Machine/6(LKASM_stFaultCSyn)
  LLStateDet_bsInInfoSyn/1 -> LL State Machine Conditions (LLSMCon)/2(LLSMCon_bsInInfoSyn)
  LLStateDet_bsLKAInPInfo/1 -> LL State Machine Conditions (LLSMCon)/3(LLSMCon_bsLKAInPInfo)
  LLStateDet_stDACMode/1 -> LL State Machine Conditions (LLSMCon)/1(LLSMCon_stDACModeIn)
  LLStateDet_stExitFlg/1 -> Delay/1
  LLStateDet_bsLLSMConClb/1 -> LL State Machine Conditions (LLSMCon)/4(LLSMCon_bsLLSMConClb)
  Delay/1 -> LL State Machine Conditions (LLSMCon)/6(LLSMCon_stExitFlg)
  LLStateDet_SignalFault/1 -> LL State Machine Conditions (LLSMCon)/7(LLSMCon_bsSignalFault)

== system LKAS_AutoSave_20200908_1055/LKAS/LL/LLOn/LL_Mon ==
  LKAMon : Inport
  Bus : BusCreator  Inputs=3
  BusInP : BusCreator  Inputs=2
  BusState : BusCreator  Inputs=2
  LLMon : Outport
  wires:
  [InPMon] -> Bus/1
  [StateMon] -> Bus/2
  LKAMon/1 -> Bus/3
  Bus/1 -> LLMon/1  "LLMon"
  [LFTTTLC_Mon] -> BusInP/1  "LFTTTLC_Mon"
  [RGTTTLC_Mon] -> BusInP/2  "RGTTTLC_Mon"
  [LDW_State_Mon] -> BusState/1  "LDW_State_Mon"
  [LKA_State_Mon] -> BusState/2  "LKA_State_Mon"
  BusInP/1 -> [InPMon]  "InPMon"
  BusState/1 -> [StateMon]  "StateMon"

== system LKAS_AutoSave_20200908_1055/LKAS/LLClb/LLSMConClb/ICv to v ==
  In1 : Inport
  Add : Sum  Inputs=+-
  Constant : Constant  Value=2.5  OutDataTypeStr=single
  Gain : Gain  Gain=1/1.02
  Out1 : Outport
  wires:
  In1/1 -> Add/1
  Add/1 -> Gain/1
  Constant/1 -> Add/2
  Gain/1 -> Out1/1

== system LKAS_AutoSave_20200908_1055/LKAS/LLClb/LLSMConClb/ICv to v1 ==
  In1 : Inport
  Add : Sum  Inputs=+-
  Constant : Constant  Value=2.5  OutDataTypeStr=single
  Gain : Gain  Gain=1/1.02
  Out1 : Outport
  wires:
  Gain/1 -> Out1/1
  Constant/1 -> Add/2
  Add/1 -> Gain/1
  In1/1 -> Add/1

== system LKAS_AutoSave_20200908_1055/LKAS/LLClb/LLSMConClb/ICv to v2 ==
  In1 : Inport
  Add : Sum  Inputs=+-
  Constant : Constant  Value=2.5  OutDataTypeStr=single
  Gain : Gain  Gain=1/1.02
  Out1 : Outport
  wires:
  In1/1 -> Add/1
  Add/1 -> Gain/1
  Constant/1 -> Add/2
  Gain/1 -> Out1/1

== system LKAS_AutoSave_20200908_1055/LKAS/LLClb/LLSMConClb/ICv to v3 ==
  In1 : Inport
  Add : Sum  Inputs=+-
  Constant : Constant  Value=2.5  OutDataTypeStr=single
  Gain : Gain  Gain=1/1.02
  Out1 : Outport
  wires:
  Gain/1 -> Out1/1
  Constant/1 -> Add/2
  Add/1 -> Gain/1
  In1/1 -> Add/1

== system LKAS_AutoSave_20200908_1055/LKAS/LLClb/LLSMConClb/ICv to v4 ==
  In1 : Inport
  Add : Sum  Inputs=+-
  Constant : Constant  Value=2.5  OutDataTypeStr=single
  Gain : Gain  Gain=1/1.02
  Out1 : Outport
  wires:
  In1/1 -> Add/1
  Add/1 -> Gain/1
  Constant/1 -> Add/2
  Gain/1 -> Out1/1

== system LKAS_AutoSave_20200908_1055/LKAS/LLClb/LLSMConClb/ICv to v5 ==
  In1 : Inport
  Add : Sum  Inputs=+-
  Constant : Constant  Value=2.5  OutDataTypeStr=single
  Gain : Gain  Gain=1/1.02
  Out1 : Outport
  wires:
  Gain/1 -> Out1/1
  Constant/1 -> Add/2
  Add/1 -> Gain/1
  In1/1 -> Add/1

== system LKAS_AutoSave_20200908_1055/LKAS/LL/Human Machine Interface (HMI)/Subsystem/Count 10s ==
  Enable : EnablePort  StatesWhenEnabling=reset
  Add : Sum
  Compare To Constant27 : simulink/Logic and Bit Operations/Compare To Constant  relop=>=  const=1000  OutDataTypeStr=boolean
  Constant : Constant  OutDataTypeStr=uint16
  Memory : Memory  InheritSampleTime=on
  Saturation : Saturate  UpperLimit=2100  LowerLimit=0
  Out : Outport  OutputWhenDisabled=reset  InitialOutput=0
  wires:
  Memory/1 -> Add/2
  Saturation/1 -> Memory/1, Compare To Constant27/1
  Add/1 -> Saturation/1
  Constant/1 -> Add/1
  Compare To Constant27/1 -> Out/1

== system LKAS_AutoSave_20200908_1055/LKAS/LL/Human Machine Interface (HMI)/Subsystem/Count 15s ==
  Enable : EnablePort  StatesWhenEnabling=reset
  Add : Sum
  Compare To Constant27 : simulink/Logic and Bit Operations/Compare To Constant  relop=>=  const=1500  OutDataTypeStr=boolean
  Constant : Constant  OutDataTypeStr=uint16
  Memory : Memory  InheritSampleTime=on
  Saturation : Saturate  UpperLimit=2100  LowerLimit=0
  Out : Outport  OutputWhenDisabled=reset  InitialOutput=0
  wires:
  Compare To Constant27/1 -> Out/1
  Constant/1 -> Add/1
  Add/1 -> Saturation/1
  Saturation/1 -> Compare To Constant27/1, Memory/1
  Memory/1 -> Add/2

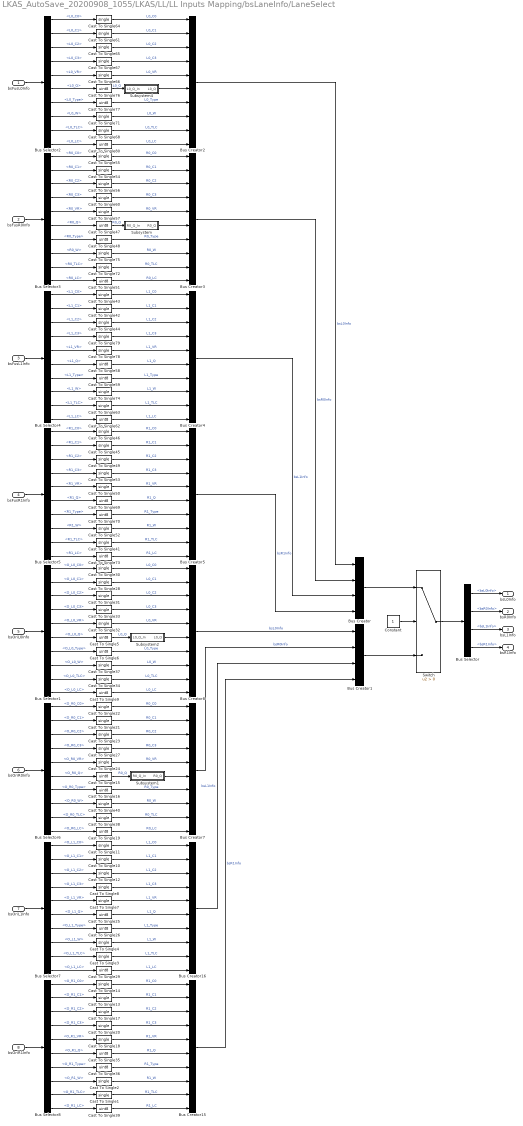
== system LKAS_AutoSave_20200908_1055/LKAS/LL/LL Inputs Mapping/bsLaneInfo/LaneSelect ==
  bsFusL0Info : Inport
  bsFusR0Info : Inport  Port=2
  bsFusL1Info : Inport  Port=3
  bsFusR1Info : Inport  Port=4
  bsOriL0Info : Inport  Port=5
  bsOriR0Info : Inport  Port=6
  bsOriL1Info : Inport  Port=7
  bsOriR1Info : Inport  Port=8
  Bus Creator : BusCreator  Inputs=4
  Bus Creator1 : BusCreator  Inputs=4
  Bus Creator{2..5,7..8,15..16} (8 alike) : BusCreator  Inputs=10
  Bus Selector : BusSelector  OutputSignals=bsL0Info,bsR0Info,bsL1Info,bsR1Info
  Bus Selector1 : BusSelector  OutputSignals=O_L0_C0,O_L0_C1,O_L0_C2,O_L0_C3,O_L0_VR,O_L0_Q,O_L0_Type,O_L0_W,O_L0_TLC,O_L0_LC
  Bus Selector2 : BusSelector  OutputSignals=L0_C0,L0_C1,L0_C2,L0_C3,L0_VR,L0_Q,L0_Type,L0_W,L0_TLC,L0_LC
  Bus Selector3 : BusSelector  OutputSignals=R0_C0,R0_C1,R0_C2,R0_C3,R0_VR,R0_Q,R0_Type,R0_W,R0_TLC,R0_LC
  Bus Selector4 : BusSelector  OutputSignals=L1_C0,L1_C1,L1_C2,L1_C3,L1_VR,L1_Q,L1_Type,L1_W,L1_TLC,L1_LC
  Bus Selector5 : BusSelector  OutputSignals=R1_C0,R1_C1,R1_C2,R1_C3,R1_VR,R1_Q,R1_Type,R1_W,R1_TLC,R1_LC
  Bus Selector6 : BusSelector  OutputSignals=O_R0_C0,O_R0_C1,O_R0_C2,O_R0_C3,O_R0_VR,O_R0_Q,O_R0_Type,O_R0_W,O_R0_TLC,O_R0_LC
  Bus Selector7 : BusSelector  OutputSignals=O_L1_C0,O_L1_C1,O_L1_C2,O_L1_C3,O_L1_VR,O_L1_Q,O_L1_Type,O_L1_W,O_L1_TLC,O_L1_LC
  Bus Selector8 : BusSelector  OutputSignals=O_R1_C0,O_R1_C1,O_R1_C2,O_R1_C3,O_R1_VR,O_R1_Q,O_R1_Type,O_R1_W,O_R1_TLC,O_R1_LC
  Cast To Single{1..4,7..8,10..14,17..18,20..24,27..28,30..34,37..38,40..46,49..50,52..57,60..61,63..68,71..72,74..75,78..79} (56 alike) : DataTypeConversion  OutDataTypeStr=single
  Cast To Single{5..6,9,15..16,19,25..26,29,35..36,39,47..48,51,58..59,62,69..70,73,76..77,80} (24 alike) : DataTypeConversion  OutDataTypeStr=uint8
  Constant : Constant  OutDataTypeStr=uint8
  Subsystem : Subsystem
  Subsystem1 : Subsystem
  Subsystem2 : Subsystem
  Subsystem4 : Subsystem
  Switch : Switch  Criteria=u2 > Threshold
  bsL0Info : Outport
  bsR0Info : Outport  Port=2
  bsL1Info : Outport  Port=3
  bsR1Info : Outport  Port=4
  wires:
  Subsystem1/1(R0_Q) -> Bus Creator7/6
  Subsystem2/1(L0_Q) -> Bus Creator8/6
  Bus Selector/4 -> bsR1Info/1  "<bsR1Info>"
  Bus Selector/3 -> bsL1Info/1  "<bsL1Info>"
  Bus Selector/2 -> bsR0Info/1  "<bsR0Info>"
  Bus Selector/1 -> bsL0Info/1  "<bsL0Info>"
  Bus Selector4/3 -> Cast To Single44/1  "<L1_C2>"
  Bus Selector4/8 -> Cast To Single74/1  "<L1_W>"
  Bus Selector5/3 -> Cast To Single49/1  "<R1_C2>"
  Bus Selector5/2 -> Cast To Single45/1  "<R1_C1>"
  Bus Selector5/8 -> Cast To Single52/1  "<R1_W>"
  Bus Creator5/1 -> Bus Creator/4  "bsR1Info"
  Bus Selector5/4 -> Cast To Single53/1  "<R1_C3>"
  Bus Selector5/9 -> Cast To Single41/1  "<R1_TLC>"
  Bus Selector3/6 -> Cast To Single47/1  "<R0_Q>"
  Subsystem/1(R0_Q) -> Bus Creator3/6
  Bus Selector2/7 -> Cast To Single77/1  "<L0_Type>"
  Bus Selector4/9 -> Cast To Single63/1  "<L1_TLC>"
  Bus Selector4/6 -> Cast To Single58/1  "<L1_Q>"
  Bus Selector4/4 -> Cast To Single79/1  "<L1_C3>"
  Bus Selector2/2 -> Cast To Single61/1  "<L0_C1>"
  Bus Selector3/1 -> Cast To Single55/1  "<R0_C0>"
  Bus Selector3/2 -> Cast To Single54/1  "<R0_C1>"
  Bus Selector2/8 -> Cast To Single71/1  "<L0_W>"
  Bus Selector3/4 -> Cast To Single60/1  "<R0_C3>"
  Bus Selector4/10 -> Cast To Single62/1  "<L1_LC>"
  Bus Selector2/1 -> Cast To Single64/1  "<L0_C0>"
  Bus Selector2/5 -> Cast To Single66/1  "<L0_VR>"
  Bus Selector5/5 -> Cast To Single50/1  "<R1_VR>"
  Bus Selector5/6 -> Cast To Single69/1  "<R1_Q>"
  Bus Selector2/9 -> Cast To Single68/1  "<L0_TLC>"
  Bus Selector5/7 -> Cast To Single70/1  "<R1_Type>"
  Bus Selector2/10 -> Cast To Single80/1  "<L0_LC>"
  Bus Selector3/3 -> Cast To Single56/1  "<R0_C2>"
  Bus Selector3/9 -> Cast To Single72/1  "<R0_TLC>"
  Bus Selector3/7 -> Cast To Single48/1  "<R0_Type>"
  Bus Selector3/8 -> Cast To Single75/1  "<R0_W>"
  Bus Selector5/1 -> Cast To Single46/1  "<R1_C0>"
  Bus Selector2/3 -> Cast To Single65/1  "<L0_C2>"
  Bus Selector5/10 -> Cast To Single73/1  "<R1_LC>"
  Bus Selector3/10 -> Cast To Single51/1  "<R0_LC>"
  bsFusL0Info/1 -> Bus Selector2/1
  Bus Selector4/7 -> Cast To Single59/1  "<L1_Type>"
  bsFusR0Info/1 -> Bus Selector3/1
  bsFusL1Info/1 -> Bus Selector4/1
  bsFusR1Info/1 -> Bus Selector5/1
  Bus Selector2/6 -> Cast To Single76/1  "<L0_Q>"
  Bus Selector2/4 -> Cast To Single67/1  "<L0_C3>"
  Bus Selector4/1 -> Cast To Single43/1  "<L1_C0>"
  Subsystem4/1(L0_Q) -> Bus Creator2/6
  Bus Selector3/5 -> Cast To Single57/1  "<R0_VR>"
  Bus Selector4/2 -> Cast To Single42/1  "<L1_C1>"
  Bus Selector4/5 -> Cast To Single78/1  "<L1_VR>"
  Switch/1 -> Bus Selector/1
  Constant/1 -> Switch/2
  Bus Creator1/1 -> Switch/3
  Bus Creator/1 -> Switch/1
  Bus Creator4/1 -> Bus Creator/3  "bsL1Info"
  Bus Creator3/1 -> Bus Creator/2  "bsR0Info"
  Bus Creator2/1 -> Bus Creator/1  "bsL0Info"
  Bus Selector8/10 -> Cast To Single39/1  "<O_R1_LC>"
  Bus Selector8/9 -> Cast To Single1/1  "<O_R1_TLC>"
  Bus Selector8/8 -> Cast To Single2/1  "<O_R1_W>"
  Bus Selector8/7 -> Cast To Single36/1  "<O_R1_Type>"
  Bus Selector8/6 -> Cast To Single35/1  "<O_R1_Q>"
  Bus Selector8/5 -> Cast To Single18/1  "<O_R1_VR>"
  Bus Selector8/4 -> Cast To Single20/1  "<O_R1_C3>"
  Bus Selector8/3 -> Cast To Single17/1  "<O_R1_C2>"
  Bus Selector8/2 -> Cast To Single13/1  "<O_R1_C1>"
  Bus Selector8/1 -> Cast To Single14/1  "<O_R1_C0>"
  bsOriR1Info/1 -> Bus Selector8/1
  Bus Selector7/10 -> Cast To Single29/1  "<O_L1_LC>"
  Bus Selector7/9 -> Cast To Single3/1  "<O_L1_TLC>"
  Bus Selector7/8 -> Cast To Single4/1  "<O_L1_W>"
  Bus Selector7/7 -> Cast To Single26/1  "<O_L1_Type>"
  Bus Selector7/6 -> Cast To Single25/1  "<O_L1_Q>"
  Bus Selector7/5 -> Cast To Single7/1  "<O_L1_VR>"
  Bus Selector7/4 -> Cast To Single8/1  "<O_L1_C3>"
  Bus Selector7/3 -> Cast To Single12/1  "<O_L1_C2>"
  Bus Selector7/2 -> Cast To Single10/1  "<O_L1_C1>"
  Bus Selector7/1 -> Cast To Single11/1  "<O_L1_C0>"
  bsOriL1Info/1 -> Bus Selector7/1
  Bus Selector6/10 -> Cast To Single19/1  "<O_R0_LC>"
  Bus Selector6/9 -> Cast To Single38/1  "<O_R0_TLC>"
  Bus Selector6/8 -> Cast To Single40/1  "<O_R0_W>"
  Bus Selector6/7 -> Cast To Single16/1  "<O_R0_Type>"
  Bus Selector6/6 -> Cast To Single15/1  "<O_R0_Q>"
  Bus Selector6/5 -> Cast To Single24/1  "<O_R0_VR>"
  Bus Selector6/4 -> Cast To Single27/1  "<O_R0_C3>"
  Bus Selector6/3 -> Cast To Single23/1  "<O_R0_C2>"
  Bus Selector6/2 -> Cast To Single21/1  "<O_R0_C1>"
  Bus Selector6/1 -> Cast To Single22/1  "<O_R0_C0>"
  bsOriR0Info/1 -> Bus Selector6/1
  Bus Selector1/10 -> Cast To Single9/1  "<O_L0_LC>"
  Bus Selector1/9 -> Cast To Single34/1  "<O_L0_TLC>"
  Bus Selector1/8 -> Cast To Single37/1  "<O_L0_W>"
  Bus Selector1/7 -> Cast To Single6/1  "<O_L0_Type>"
  Bus Selector1/6 -> Cast To Single5/1  "<O_L0_Q>"
  Bus Selector1/5 -> Cast To Single32/1  "<O_L0_VR>"
  Bus Selector1/4 -> Cast To Single33/1  "<O_L0_C3>"
  Bus Selector1/3 -> Cast To Single31/1  "<O_L0_C2>"
  Bus Selector1/2 -> Cast To Single28/1  "<O_L0_C1>"
  Bus Selector1/1 -> Cast To Single30/1  "<O_L0_C0>"
  bsOriL0Info/1 -> Bus Selector1/1
  Cast To Single2/1 -> Bus Creator15/8  "R1_W"
  Cast To Single27/1 -> Bus Creator7/4  "R0_C3"
  Cast To Single10/1 -> Bus Creator16/2  "L1_C1"
  Cast To Single32/1 -> Bus Creator8/5  "L0_VR"
  Cast To Single37/1 -> Bus Creator8/8  "L0_W"
  Cast To Single40/1 -> Bus Creator7/8  "R0_W"
  Bus Creator8/1 -> Bus Creator1/1  "bsL0Info"
  Cast To Single22/1 -> Bus Creator7/1  "R0_C0"
  Cast To Single25/1 -> Bus Creator16/6  "L1_Q"
  Cast To Single17/1 -> Bus Creator15/3  "R1_C2"
  Cast To Single36/1 -> Bus Creator15/7  "R1_Type"
  Cast To Single9/1 -> Bus Creator8/10  "L0_LC"
  Cast To Single31/1 -> Bus Creator8/3  "L0_C2"
  Cast To Single30/1 -> Bus Creator8/1  "L0_C0"
  Cast To Single33/1 -> Bus Creator8/4  "L0_C3"
  Cast To Single5/1 -> Subsystem2/1(L0_Q_In)  "L0_Q"
  Cast To Single6/1 -> Bus Creator8/7  "L0_Type"
  Cast To Single16/1 -> Bus Creator7/7  "R0_Type"
  Cast To Single35/1 -> Bus Creator15/6  "R1_Q"
  Cast To Single28/1 -> Bus Creator8/2  "L0_C1"
  Cast To Single1/1 -> Bus Creator15/9  "R1_TLC"
  Cast To Single21/1 -> Bus Creator7/2  "R0_C1"
  Cast To Single23/1 -> Bus Creator7/3  "R0_C2"
  Bus Creator16/1 -> Bus Creator1/3  "bsL1Info"
  Cast To Single13/1 -> Bus Creator15/2  "R1_C1"
  Cast To Single14/1 -> Bus Creator15/1  "R1_C0"
  Cast To Single26/1 -> Bus Creator16/7  "L1_Type"
  Cast To Single20/1 -> Bus Creator15/4  "R1_C3"
  Cast To Single24/1 -> Bus Creator7/5  "R0_VR"
  Cast To Single7/1 -> Bus Creator16/5  "L1_VR"
  Cast To Single15/1 -> Subsystem1/1(R0_Q_In)  "R0_Q"
  Cast To Single11/1 -> Bus Creator16/1  "L1_C0"
  Cast To Single38/1 -> Bus Creator7/9  "R0_TLC"
  Cast To Single4/1 -> Bus Creator16/8  "L1_W"
  Cast To Single12/1 -> Bus Creator16/3  "L1_C2"
  Cast To Single19/1 -> Bus Creator7/10  "R0_LC"
  Cast To Single39/1 -> Bus Creator15/10  "R1_LC"
  Cast To Single18/1 -> Bus Creator15/5  "R1_VR"
  Cast To Single3/1 -> Bus Creator16/9  "L1_TLC"
  Cast To Single29/1 -> Bus Creator16/10  "L1_LC"
  Cast To Single8/1 -> Bus Creator16/4  "L1_C3"
  Bus Creator15/1 -> Bus Creator1/4  "bsR1Info"
  Cast To Single34/1 -> Bus Creator8/9  "L0_TLC"
  Bus Creator7/1 -> Bus Creator1/2  "bsR0Info"
  Cast To Single61/1 -> Bus Creator2/2  "L0_C1"
  Cast To Single66/1 -> Bus Creator2/5  "L0_VR"
  Cast To Single67/1 -> Bus Creator2/4  "L0_C3"
  Cast To Single65/1 -> Bus Creator2/3  "L0_C2"
  Cast To Single64/1 -> Bus Creator2/1  "L0_C0"
  Cast To Single76/1 -> Subsystem4/1(L0_Q_In)  "L0_Q"
  Cast To Single68/1 -> Bus Creator2/9  "L0_TLC"
  Cast To Single77/1 -> Bus Creator2/7  "L0_Type"
  Cast To Single80/1 -> Bus Creator2/10  "L0_LC"
  Cast To Single56/1 -> Bus Creator3/3  "R0_C2"
  Cast To Single54/1 -> Bus Creator3/2  "R0_C1"
  Cast To Single55/1 -> Bus Creator3/1  "R0_C0"
  Cast To Single47/1 -> Subsystem/1(R0_Q_In)  "R0_Q"
  Cast To Single48/1 -> Bus Creator3/7  "R0_Type"
  Cast To Single51/1 -> Bus Creator3/10  "R0_LC"
  Cast To Single57/1 -> Bus Creator3/5  "R0_VR"
  Cast To Single60/1 -> Bus Creator3/4  "R0_C3"
  Cast To Single72/1 -> Bus Creator3/9  "R0_TLC"
  Cast To Single75/1 -> Bus Creator3/8  "R0_W"
  Cast To Single44/1 -> Bus Creator4/3  "L1_C2"
  Cast To Single58/1 -> Bus Creator4/6  "L1_Q"
  Cast To Single59/1 -> Bus Creator4/7  "L1_Type"
  Cast To Single43/1 -> Bus Creator4/1  "L1_C0"
  Cast To Single42/1 -> Bus Creator4/2  "L1_C1"
  Cast To Single78/1 -> Bus Creator4/5  "L1_VR"
  Cast To Single79/1 -> Bus Creator4/4  "L1_C3"
  Cast To Single62/1 -> Bus Creator4/10  "L1_LC"
  Cast To Single63/1 -> Bus Creator4/9  "L1_TLC"
  Cast To Single74/1 -> Bus Creator4/8  "L1_W"
  Cast To Single45/1 -> Bus Creator5/2  "R1_C1"
  Cast To Single46/1 -> Bus Creator5/1  "R1_C0"
  Cast To Single49/1 -> Bus Creator5/3  "R1_C2"
  Cast To Single50/1 -> Bus Creator5/5  "R1_VR"
  Cast To Single52/1 -> Bus Creator5/8  "R1_W"
  Cast To Single53/1 -> Bus Creator5/4  "R1_C3"
  Cast To Single41/1 -> Bus Creator5/9  "R1_TLC"
  Cast To Single69/1 -> Bus Creator5/6  "R1_Q"
  Cast To Single70/1 -> Bus Creator5/7  "R1_Type"
  Cast To Single73/1 -> Bus Creator5/10  "R1_LC"
  Cast To Single71/1 -> Bus Creator2/8  "L0_W"

== system LKAS_AutoSave_20200908_1055/LKAS/LL/LL Inputs Mapping/bsLaneInfo/LanesReconstruct  ==
  bsL0Info : Inport
  bsR0Info : Inport  Port=2
  bsL1Info : Inport  Port=3
  bsR1Info : Inport  Port=4
  Bus Selector5 : BusSelector  OutputSignals=L0_Q
  Bus Selector6 : BusSelector  OutputSignals=R0_Q
  LaneReconstructSM : Stateflow chart  TreatAsAtomicUnit=on
  Left 1Lane Reconstruct (Lft1LaneR) : Subsystem
  Left Lane Reconstruct (LftLaneR) : Subsystem
  Right 1Lane Reconstruct (Rgt1LaneR) : Subsystem
  Right Lane Reconstruct (RgtLaneR) : Subsystem
  RoadSide Offset : Subsystem
  Switch : Switch  Criteria=u2 > Threshold
  Switch1 : Switch  Criteria=u2 > Threshold
  bsL0InfoR : Outport
  bsR0InfoR : Outport  Port=2
  bsL1InfoR : Outport  Port=3
  bsR1InfoR : Outport  Port=4
  wires:
  bsL1Info/1 -> Left 1Lane Reconstruct (Lft1LaneR)/2(bsL1Info)
  Bus Selector6/1 -> LaneReconstructSM/2(LaneRSM_stR0Ql)  "<R0_Q>"
  Bus Selector5/1 -> LaneReconstructSM/1(LaneRSM_stL0Ql)  "<L0_Q>"
  RoadSide Offset/3(lRoadW) -> [RoadWidth], Left Lane Reconstruct (LftLaneR)/1(lRoadW), Right Lane Reconstruct (RgtLaneR)/3(lRoadW)
  Left Lane Reconstruct (LftLaneR)/1(bsL0InfoR) -> Switch1/3
  Right Lane Reconstruct (RgtLaneR)/1(bsR0InfoR) -> Switch/3
  Switch/1 -> bsR0InfoR/1
  Switch1/1 -> bsL0InfoR/1
  LaneReconstructSM/1(LaneRSM_stRoadFlg) -> [RoadFlg]
  LaneReconstructSM/2(LaneRSM_stLftFlg) -> [LftFlg]
  LaneReconstructSM/3(LaneRSM_stRgtFlg) -> [RgtFlg]
  bsR1Info/1 -> Right 1Lane Reconstruct (Rgt1LaneR)/2(bsR1Info)
  Right 1Lane Reconstruct (Rgt1LaneR)/1(bsL1InfoR) -> bsR1InfoR/1
  Left 1Lane Reconstruct (Lft1LaneR)/1(bsL1InfoR) -> bsL1InfoR/1
  [RgtFlg] -> Right 1Lane Reconstruct (Rgt1LaneR)/1(stFlag)
  [LftFlg] -> Left 1Lane Reconstruct (Lft1LaneR)/1(stFlag)
  [RgtFlg] -> Switch/2
  [LftFlg] -> Switch1/2
  bsR0Info/1 -> RoadSide Offset/2(bsR0Info)
  bsL0Info/1 -> RoadSide Offset/1(bsL0Info)
  RoadSide Offset/1(bsL0Infoout) -> Left Lane Reconstruct (LftLaneR)/3(bsL0Info), Switch1/1, Right Lane Reconstruct (RgtLaneR)/1(bsL0Info), Bus Selector5/1
  RoadSide Offset/2(bsR0Infoout) -> Switch/1, Right Lane Reconstruct (RgtLaneR)/2(bsR0Info), Left Lane Reconstruct (LftLaneR)/2(bsR0Info), Bus Selector6/1

== system LKAS_AutoSave_20200908_1055/LKAS/LL/LLOn/LDW/Heading Angle Detection (HdAgDet) ==
  HdAgDet_stLDWActvFlg : Inport
  HdAgDet_phiHdAgLft : Inport  Port=2
  HdAgDet_phiHdAgRgt : Inport  Port=3
  HdAgDet_phiHdAgThres_C : Inport  Port=4
  Constant : Constant  Value=5  OutDataTypeStr=single
  If : If  IfExpression=u1==1  ElseIfExpressions=u1==2
  If Action Subsystem : Subsystem  TreatAsAtomicUnit=on
  If Action Subsystem1 : Subsystem  TreatAsAtomicUnit=on
  If Action Subsystem2 : Subsystem  TreatAsAtomicUnit=on
  Merge : Merge  Inputs=3  InitialOutput=0
  Relational Operator : RelationalOperator  OutDataTypeStr=boolean  RndMeth=Nearest
  Sum Condition : Subsystem
  HdAgDet_stHdAgDetFlg : Outport
  wires:
  If/1 -> If Action Subsystem/Action
  If Action Subsystem/1(Out1) -> Merge/1
  If Action Subsystem1/1(Out1) -> Merge/2
  If/2 -> If Action Subsystem1/Action
  If Action Subsystem2/1(Out1) -> Merge/3
  If/3 -> If Action Subsystem2/Action
  HdAgDet_phiHdAgLft/1 -> If Action Subsystem/1(In1)
  HdAgDet_phiHdAgRgt/1 -> If Action Subsystem1/1(In1)
  HdAgDet_stLDWActvFlg/1 -> If/1
  Merge/1 -> Relational Operator/1
  HdAgDet_phiHdAgThres_C/1 -> Relational Operator/2
  Sum Condition/1(Out) -> HdAgDet_stHdAgDetFlg/1
  Relational Operator/1 -> Sum Condition/1(In), Sum Condition/Enable
  Constant/1 -> Sum Condition/2(Sum)

== system LKAS_AutoSave_20200908_1055/LKAS/LL/LLOn/LKA/Driver Torque Addition (DTA) ==
  DTA_bsInInfoSyn : Inport
  DTA_bsLFClb : Inport  Port=2
  Bus Selector : BusSelector  OutputSignals=LL_LKASWAClb.LL_LKASWASyn_TrqSwaAddSwt
  Compare To Constant : simulink/Logic and Bit Operations/Compare To Constant  relop=>  const=0  OutDataTypeStr=boolean
  Subsystem : Subsystem
  Subsystem1 : Subsystem
  DTA_phiDTASWACmd : Outport
  DTA_M : Outport  Port=2
  wires:
  [LKA_SampleTime] -> Subsystem/3(LKA_SampleTime)
  DTA_bsInInfoSyn/1 -> Subsystem/1(DTA_bsInInfoSyn), Subsystem1/1(DTA_bsInInfoSyn)
  DTA_bsLFClb/1 -> Subsystem1/2(DTA_bsLFClb), Subsystem/2(DTA_bsLFClb), Bus Selector/1
  Subsystem/1(Out1) -> DTA_phiDTASWACmd/1
  Subsystem1/1(Out1) -> DTA_M/1
  Bus Selector/1 -> Compare To Constant/1  "<LL_LKASWASyn_TrqSwaAddSwt>"
  Compare To Constant/1 -> Subsystem/Enable

== system LKAS_AutoSave_20200908_1055/LKAS/LL/LLOn/LKA/LKA Exit Processing (LKAExPrcs) ==
  LKAExPrcs_bsInInfoSyn : Inport
  LKAExPrcs_bsLKAInPInfo : Inport  Port=2
  LKAExPrcs_bsLKAClb : Inport  Port=3
  LKAExPrcs_PlanT1 : Inport  Port=4
  Cast To Single : DataTypeConversion  OutDataTypeStr=single
  Exit Time 1 : Subsystem
  Exit Time 2 : Subsystem
  Exit Time 3 : Subsystem
  Fcn : Fcn  Expr=u(3)*(u(3)==1)*3+u(2)*(u(3)==0)*2+u(1)*(u(2)==0&&u(3)==0)
  Logical Operator3 : Logic  Operator=OR  Inputs=3  AllPortsSameDT=off  OutDataTypeStr=boolean
  Mux : Mux  Inputs=3
  LKAExPrcs_stExFlg : Outport
  LKAExPrcs_stExNum : Outport  Port=2
  wires:
  LKAExPrcs_bsInInfoSyn/1 -> Exit Time 3/1(bsInInfoSyn), Exit Time 2/1(bsInInfoSyn)
  Logical Operator3/1 -> LKAExPrcs_stExFlg/1
  Exit Time 1/1(Exit1) -> Mux/1, Logical Operator3/1
  Exit Time 2/1(Exit2) -> Mux/2, Logical Operator3/2
  Exit Time 3/1(Exit3) -> Mux/3, Logical Operator3/3
  LKAExPrcs_bsLKAInPInfo/1 -> Exit Time 3/2(bsLKAInPInfo), Exit Time 2/3(bsLKAInPInfo), Exit Time 1/1(bsLKAInPInfo)
  LKAExPrcs_bsLKAClb/1 -> Exit Time 1/2(bsLKAClb), Exit Time 2/2(bsLKAClb), Exit Time 3/3(bsLKAClb)
  LKAExPrcs_PlanT1/1 -> Exit Time 2/4(T1), Exit Time 3/4(T1)
  Mux/1 -> Cast To Single/1
  Fcn/1 -> LKAExPrcs_stExNum/1  "ExNum"
  Cast To Single/1 -> Fcn/1
